simulink model "Studio10b_tune"  (R2017b)
settings: Solver=ode45  StartTime=0.  StopTime=60  FixedStep=0.2  MaxStep=0.05  RelTol=1e-8  AbsTol=1e-8  EnableMultiTasking=on
settings Model: ExtModeTrigMode=oneshot  ExtModeArmWhenConnect=off  Creator=LEVIENKL  LastModifiedBy=carlislt
settings DataIOCC: SaveFormat=Array  SignalLoggingSaveFormat=ModelDataLogs  SaveOutput=off  SaveTime=off  SignalLoggingName=sigsOut
settings OptimizationCC: BlockReduction=off  BooleanDataType=off  ExpressionDepthLimit=2147483647  InitFltsAndDblsToZero=on  LifeSpan=inf
settings DebuggingCC: SaveWithParameterizedLinksMsg=none  UnderspecifiedInitializationDetection=Classic  MergeDetectMultiDrivingBlocksExec=none  SignalResolutionControl=TryResolveAllWithWarning  MultiTaskDSMMsg=warning  MultiTaskCondExecSysMsg=none  FcnCallInpInsideContextMsg=warning  AllowSymbolicDim=off  StateNameClashWarn=warning  SFUnexpectedBacktrackingDiag=warning  SFNoUnconditionalDefaultTransitionDiag=warning  SFExecutionAtInitializationDiag=none
settings HardwareCC: ProdBitPerPointer=32  ProdBitPerSizeT=32  ProdBitPerPtrDiffT=32  ProdLargestAtomicFloat=None  ProdIntDivRoundTo=Undefined  ProdEndianess=Unspecified  ProdWordSize=32  ProdHWDeviceType=32-bit Generic  TargetUnknown=on
settings ModelReferenceCC: PropagateSignalLabelsOutOfModel=off
settings CodeAppCC: StateflowObjectComments=on
settings GRTTargetCC: TargetFcnLib=ansi_tfl_tmw.mat  TargetLangStandard=C89/C90 (ANSI)  GeneratePreprocessorConditionals=Disable all  CombineOutputUpdateFcns=off  GRTInterface=on
settings ConfigComp: CovMetricSettings=dw  CovHtmlReporting=on  CovSaveCumulativeToWorkspaceVar=on  CovSaveSingleToWorkspaceVar=on  CovExternalEMLEnable=off  CovSFcnEnable=off

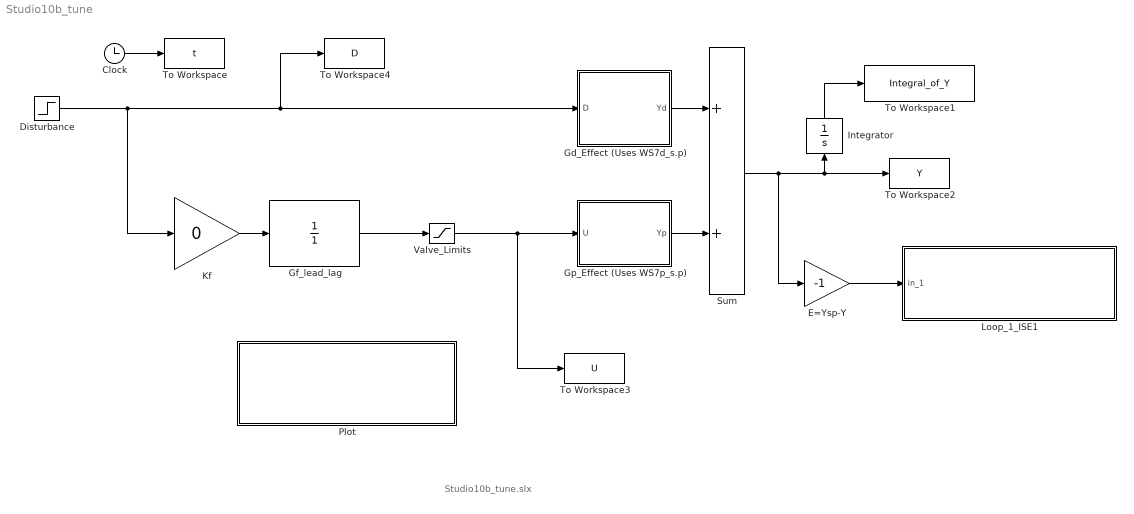
== system Studio10b_tune ==
  note: Studio10b_tune.slx
  " Integrator" : Integrator
  Clock : Clock
  Disturbance : Step  Time=5  SampleTime=0  ZeroCross=off
      settings: AttributesFormatString=%<Before> to %<After>\nat %<Time>
  E=Ysp-Y : Gain  Gain=-1  SaturateOnIntegerOverflow=on  OutDataTypeStr=Inherit: Same as input  ParamDataTypeStr=Inherit: Same as input
  Gd_Effect (Uses WS7d_s.p) : Subsystem
  Gf_lead_lag : TransferFcn  Denominator=[1]
  Gp_Effect (Uses WS7p_s.p) : Subsystem
  Kf : Gain  Gain=0  SaturateOnIntegerOverflow=on  OutDataTypeStr=Inherit: Same as input  ParamDataTypeStr=Inherit: Same as input
  Loop_1_ISE1 : Subsystem  mask(Integral Squarred Evaluation - Loop 1){}
      settings: OpenFcn=ISE1
      mask Help: This block calculates and plots loop #1 ISE.
      mask Display: disp('After Loop 1 Simulation:\n Double Click for ISE evaluation\n (uses ISE1.p)')
  Plot : Subsystem  mask(FF tuning plots){}
      settings: OpenFcn=FF_tuneP
      mask Help: This block plots FF tunig curves.
      mask Display: disp('After Simulation:\n Double Click for Plots\n (uses FF_tuneP.m)')
  Sum : Sum  SaturateOnIntegerOverflow=on  InputSameDT=on  OutDataTypeStr=Inherit: Same as first input
  To Workspace : ToWorkspace  VariableName=t  SampleTime=-1
  To Workspace1 : ToWorkspace  VariableName=Integral_of_Y  SampleTime=-1
  To Workspace2 : ToWorkspace  VariableName=Y  SampleTime=-1
  To Workspace3 : ToWorkspace  VariableName=U  SampleTime=-1
  To Workspace4 : ToWorkspace  VariableName=D  SampleTime=-1
  Valve_Limits : Saturate  UpperLimit=50  LowerLimit=-50  ZeroCross=off
      settings: AttributesFormatString=%<UpperLimit>\n%<LowerLimit>
  wires:
  Sum/1 -> E=Ysp-Y/1, To Workspace2/1, " Integrator"/1
  Gp_Effect (Uses WS7p_s.p)/1(Yp) -> Sum/2
  Valve_Limits/1 -> To Workspace3/1, Gp_Effect (Uses WS7p_s.p)/1(U)
  Gf_lead_lag/1 -> Valve_Limits/1
  Clock/1 -> To Workspace/1
  " Integrator"/1 -> To Workspace1/1
  Gd_Effect (Uses WS7d_s.p)/1(Yd) -> Sum/1
  Disturbance/1 -> Kf/1, To Workspace4/1, Gd_Effect (Uses WS7d_s.p)/1(D)
  Kf/1 -> Gf_lead_lag/1
  E=Ysp-Y/1 -> Loop_1_ISE1/1(in_1)

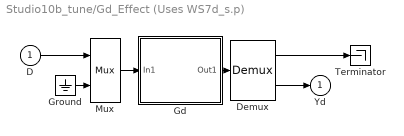
== system Studio10b_tune/Gd_Effect (Uses WS7d_s.p) ==
  D : Inport
  Demux : Demux  Outputs=2
  Gd : Subsystem  mask(Gf_tuning){}
      mask help:
      | CHE 461 Gf tuning
      | MATLAB v2014b
      | Dr. K.L. Levien
      | School of CBEE
      | Oregon State University
      | Corvallis, Oregon 97331-2702
      mask Help:
      | CHE 461 = Process Control
      | Gd for Gf tuning WS7
      | School of CBEE, Oregon State University
      mask Display: disp('Gf effect')
  Ground : Ground
  Mux : Mux  Inputs=2
  Terminator : Terminator
  Yd : Outport
  wires:
  Ground/1 -> Mux/2
  Mux/1 -> Gd/1(In1)
  Gd/1(Out1) -> Demux/1
  D/1 -> Mux/1
  Demux/1 -> Terminator/1
  Demux/2 -> Yd/1

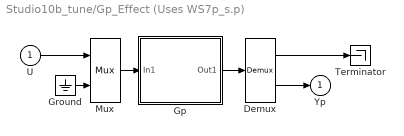
== system Studio10b_tune/Gp_Effect (Uses WS7p_s.p) ==
  U : Inport
  Demux : Demux  Outputs=2
  Gp : Subsystem  mask(Gf_tuning){}
      mask help:
      | CHE 461 Gf tuning
      | MATLAB v2014b
      | Dr. K.L. Levien
      | School of CBEE
      | Oregon State University
      | Corvallis, Oregon 97331-2702
      mask Help:
      | CHE 461 = Process Control
      | Gd for Gf tuning WS7
      | School of CBEE, Oregon State University
      mask Display: disp('Gp effect')
  Ground : Ground
  Mux : Mux  Inputs=2
  Terminator : Terminator
  Yp : Outport
  wires:
  Ground/1 -> Mux/2
  Mux/1 -> Gp/1(In1)
  Gp/1(Out1) -> Demux/1
  U/1 -> Mux/1
  Demux/1 -> Terminator/1
  Demux/2 -> Yp/1

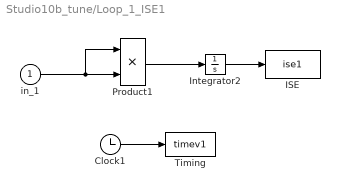
== system Studio10b_tune/Loop_1_ISE1 ==
  in_1 : Inport
  Clock1 : Clock
  ISE : ToWorkspace  VariableName=ise1
      settings: MaxDataPoints=20000
  Integrator2 : Integrator
  Product1 : Product  SaturateOnIntegerOverflow=on  RndMeth=Zero  InputSameDT=on  OutDataTypeStr=Inherit: Same as first input
  Timing : ToWorkspace  VariableName=timev1
      settings: MaxDataPoints=20000
  wires:
  in_1/1 -> Product1/2, Product1/1
  Integrator2/1 -> ISE/1
  Clock1/1 -> Timing/1
  Product1/1 -> Integrator2/1

== system Studio10b_tune/Plot ==

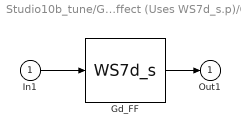
== system Studio10b_tune/Gd_Effect (Uses WS7d_s.p)/Gd ==
  In1 : Inport
  Gd_FF : S-Function  FunctionName=WS7d_s  SFunctionDeploymentMode=off  EnableBusSupport=off
  Out1 : Outport
  wires:
  In1/1 -> Gd_FF/1
  Gd_FF/1 -> Out1/1

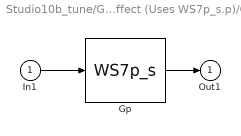
== system Studio10b_tune/Gp_Effect (Uses WS7p_s.p)/Gp ==
  In1 : Inport
  Gp : S-Function  FunctionName=WS7p_s  SFunctionDeploymentMode=off  EnableBusSupport=off
  Out1 : Outport
  wires:
  In1/1 -> Gp/1
  Gp/1 -> Out1/1
